simulink model "testing_control_with_feedback_estimate"  (Simulink 7.9)
settings: Solver=ode45  StartTime=0.0  StopTime=5  RelTol=1e-3
libraries: powerlib x6
settings Model: Creator=Dmitriy  LastModifiedBy=Dmitriy

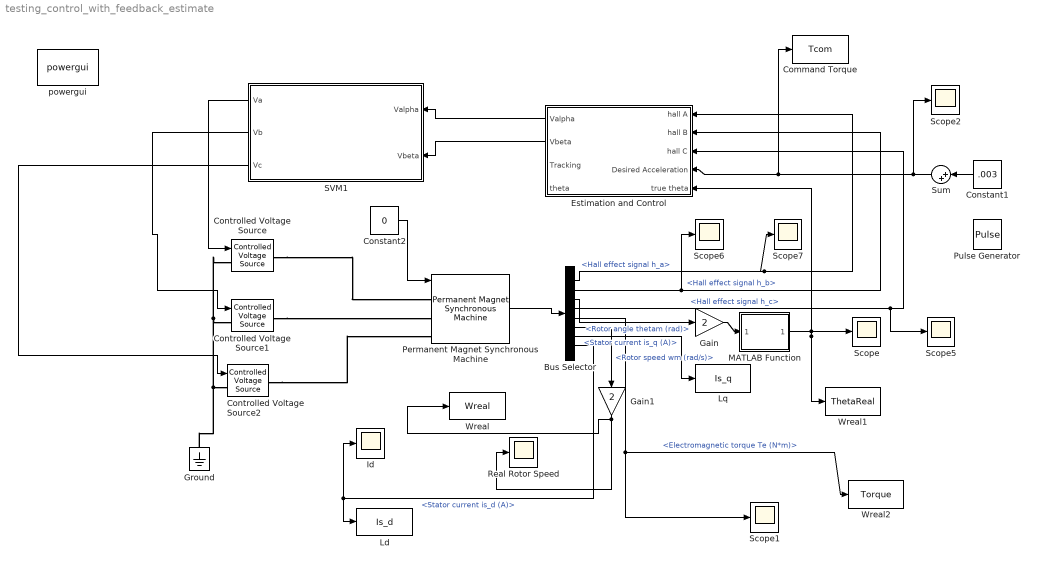
== system testing_control_with_feedback_estimate ==
  Bus Selector : BusSelector  OutputSignals=Hall effect signal h_a,Hall effect signal h_b,Hall effect signal h_c,Rotor angle thetam (rad),Electromagnetic torque Te (N*m),Rotor speed wm (rad/s),Stator current is_q (A),Stator current is_d (A)
  Command Torque : ToWorkspace  VariableName=Tcom  SampleTime=-1  SaveFormat=Timeseries
  Constant1 : Constant  Value=.003
  Constant2 : Constant  Value=0
  Controlled Voltage Source : powerlib/Electrical Sources/Controlled Voltage Source  Initialize=off  Source_Type=DC  Amplitude=0  Phase=0  Frequency=0  Measurements=None
  Controlled Voltage Source1 : powerlib/Electrical Sources/Controlled Voltage Source  Initialize=off  Source_Type=AC  Amplitude=0  Phase=0  Frequency=0  Measurements=None
  Controlled Voltage Source2 : powerlib/Electrical Sources/Controlled Voltage Source  Initialize=off  Source_Type=AC  Amplitude=0  Phase=0  Frequency=0  Measurements=None
  Estimation and Control : Subsystem  TreatAsAtomicUnit=on
  Gain : Gain  Gain=2
  Gain1 : Gain  Gain=2
  Ground : powerlib/Elements/Ground  LConnTagsString=a
  Id : Scope
      settings: YMin=-0.12  YMax=1.38778e-17  SaveName=ScopeData10
  Ld : ToWorkspace  VariableName=Is_d  SampleTime=-1  SaveFormat=Timeseries
  Lq : ToWorkspace  VariableName=Is_q  SampleTime=-1  SaveFormat=Timeseries
  MATLAB Function : MATLAB Function  TreatAsAtomicUnit=on
  Permanent Magnet Synchronous Machine : powerlib/Machines/Permanent Magnet Synchronous Machine  NbPhases=3  FluxDistribution=Sinusoidal  RotorType=Round  MechanicalLoad=Torque Tm  PresetModel=No  ShowDetailedParameters=on  Resistance=28.2  Inductance=8.5e-3  dqInductances=[0.006365 0.006365]  La=1940*10^-6  MachineConstant=Torque Constant (N.m / A_peak)  Flux=0.005225  VoltageCst=1.8954  TorqueCst=0.0181*sqrt(3)/2  Flat=120  Mechanical=[0.0001 1.35e-007 2 0]  PolePairs=2  InitialConditions=[2.5, 49.6, 0,0]  InitialConditions5ph=[0 0 0 0 0 0]  TsPowergui=0  TsBlock=-1  RefAngle=Aligned with phase A axis (original Park)
      link override From: GotoTag=tp895c948e_709d_4b9e_9e5d_f832b5ab97a5
  Pulse Generator : DiscretePulseGenerator  PulseType=Time based  Amplitude=-.006  Period=3  PulseWidth=50
  Real Rotor Speed : Scope
      settings: YMin=9.27  YMax=9.44  SaveName=ScopeData11
  SVM1 : Subsystem  TreatAsAtomicUnit=on  SystemSampleTime=.0001
  Scope{,1..2,5..7} (6 alike) : Scope
      Scope settings: YMin=0.03925  YMax=0.0396
      Scope1 settings: YMin=-1.1e+07  YMax=1.2e+07
      Scope2 settings: YMin=0.00317  YMax=0.00334  SaveName=ScopeData21
      Scope5 settings: SaveName=ScopeData5
      Scope6 settings: SaveName=ScopeData18
      Scope7 settings: SaveName=ScopeData20
  Sum : Sum  Inputs=|++
  Wreal : ToWorkspace  VariableName=Wreal  SampleTime=-1  SaveFormat=Timeseries
  Wreal1 : ToWorkspace  VariableName=ThetaReal  SampleTime=-1  SaveFormat=Timeseries
  Wreal2 : ToWorkspace  VariableName=Torque  SampleTime=-1  SaveFormat=Timeseries
  powergui : powerlib/powergui  Priority=1  SimulationMode=Continuous  SolverType=Tustin  SampleTime=50e-6  frequency=60  SPID=off  DisableSnubberDevices=off  DisableRonSwitches=off  DisableVfSwitches=off  SwTol=0  Interpol=off  DisplayEquations=off  FunctionMessages=off  frequencyindice=0  Pbase=100e6  ErrMax=1e-4  Iterations=50  UnitsV=kV  UnitsW=MW  echomessages=off  HookPort=off  EnableUseOfTLC=off  x0status=blocks  RestoreLinks=warning  ResistiveCurrentMeasurement=off  Ylog=off  Xlog=on  ShowGrid=off  save=off  variable=ZData  ZoomFFT=off  StartTime=0.0  cycles=1  DisplayStyle=1  FreqAxis=off  MaxFrequency=1000  frequencyindicesteady=1  display=off  methode=off
  wires:
  Permanent Magnet Synchronous Machine/1 -> Bus Selector/1
  Bus Selector/1 -> Estimation and Control/1(hall A), Scope7/1  "<Hall effect signal h_a>"
  Bus Selector/3 -> Estimation and Control/3(hall C), Scope5/1  "<Hall effect signal h_c>"
  Bus Selector/4 -> Gain/1  "<Rotor angle thetam (rad)>"
  Bus Selector/5 -> Wreal2/1, Scope1/1  "<Electromagnetic torque Te (N*m)>"
  Bus Selector/2 -> Estimation and Control/2(hall B), Scope6/1  "<Hall effect signal h_b>"
  Bus Selector/6 -> Gain1/1  "<Rotor speed wm (rad/s)>"
  MATLAB Function/1(lambda1) -> Wreal1/1, Scope/1, Estimation and Control/5(true theta)
  Gain/1 -> MATLAB Function/1(lambda)
  Constant2/1 -> Permanent Magnet Synchronous Machine/1
  Estimation and Control/1(Valpha) -> SVM1/1(Valpha)
  Estimation and Control/2(Vbeta) -> SVM1/2(Vbeta)
  Bus Selector/7 -> Lq/1  "<Stator current is_q (A)>"
  Bus Selector/8 -> Ld/1, Id/1  "<Stator current is_d (A)>"
  SVM1/1(Va) -> Controlled Voltage Source/1
  SVM1/2(Vb) -> Controlled Voltage Source1/1
  SVM1/3(Vc) -> Controlled Voltage Source2/1
  Constant1/1 -> Sum/1
  Sum/1 -> Scope2/1, Estimation and Control/4(Desired Acceleration), Command Torque/1
  Gain1/1 -> Real Rotor Speed/1, Wreal/1
  connections:
  Controlled Voltage Source2/LConn1 -- Controlled Voltage Source1/LConn1 -- Controlled Voltage Source/LConn1 -- Ground/LConn1
  Controlled Voltage Source/RConn1 -- Permanent Magnet Synchronous Machine/LConn1
  Controlled Voltage Source2/RConn1 -- Permanent Magnet Synchronous Machine/LConn3
  Controlled Voltage Source1/RConn1 -- Permanent Magnet Synchronous Machine/LConn2

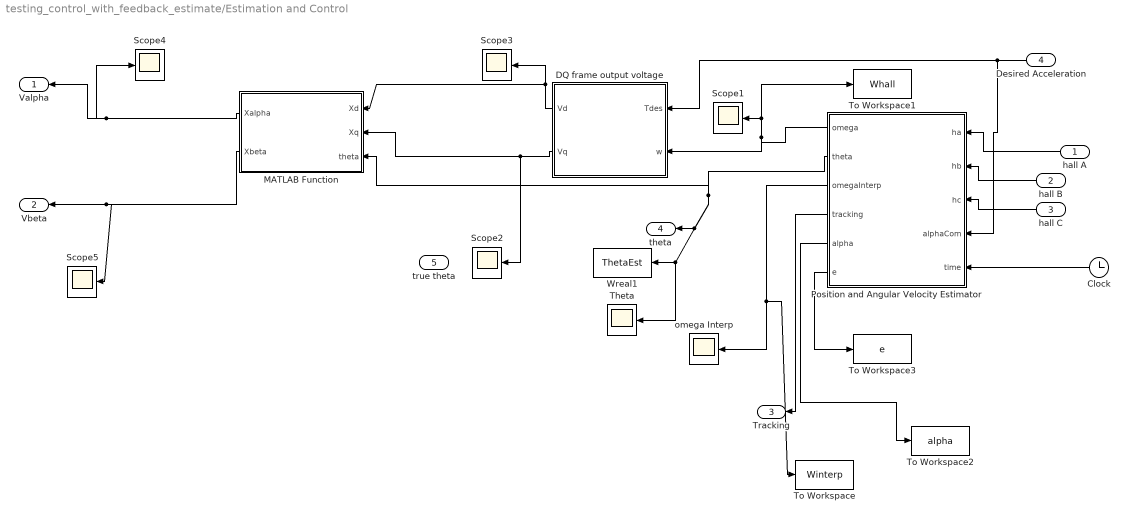
== system testing_control_with_feedback_estimate/Estimation and Control ==
  hall A : Inport
  hall B : Inport  Port=2
  hall C : Inport  Port=3
  Desired Acceleration : Inport  Port=4
  true theta : Inport  Port=5
  Clock : Clock
  DQ frame output voltage : MATLAB Function  TreatAsAtomicUnit=on
  MATLAB Function : MATLAB Function  TreatAsAtomicUnit=on
  Position and Angular Velocity Estimator : MATLAB Function  TreatAsAtomicUnit=on
  Scope{1..5} (5 alike) : Scope
      Scope1 settings: YMin=73.5  YMax=80  SaveName=ScopeData13
      Scope2 settings: YMin=4.44033  YMax=4.90773  SaveName=ScopeData14
      Scope3 settings: SaveName=ScopeData15
      Scope4 settings: SaveName=ScopeData16
      Scope5 settings: SaveName=ScopeData17
  Theta : Scope
      settings: YMin=0  YMax=6.5  SaveName=ScopeData12
  To Workspace : ToWorkspace  VariableName=Winterp  SampleTime=-1  SaveFormat=Timeseries
  To Workspace1 : ToWorkspace  VariableName=Whall  SampleTime=-1  SaveFormat=Timeseries
  To Workspace2 : ToWorkspace  VariableName=alpha  SampleTime=-1  SaveFormat=Timeseries
  To Workspace3 : ToWorkspace  VariableName=e  SampleTime=-1  SaveFormat=Timeseries
  Wreal1 : ToWorkspace  VariableName=ThetaEst  SampleTime=-1  SaveFormat=Timeseries
  omega Interp : Scope
      settings: YMin=0  YMax=3.25  SaveName=ScopeData19
  Valpha : Outport
  Vbeta : Outport  Port=2
  Tracking : Outport  Port=3
  theta : Outport  Port=4
  wires:
  Position and Angular Velocity Estimator/1(omega) -> Scope1/1, To Workspace1/1, DQ frame output voltage/2(w)
  Desired Acceleration/1 -> DQ frame output voltage/1(Tdes), Position and Angular Velocity Estimator/4(alphaCom)
  hall A/1 -> Position and Angular Velocity Estimator/1(ha)
  hall B/1 -> Position and Angular Velocity Estimator/2(hb)
  hall C/1 -> Position and Angular Velocity Estimator/3(hc)
  Position and Angular Velocity Estimator/2(theta) -> Theta/1, Wreal1/1, theta/1, MATLAB Function/3(theta)
  DQ frame output voltage/2(Vq) -> Scope2/1, MATLAB Function/2(Xq)
  DQ frame output voltage/1(Vd) -> Scope3/1, MATLAB Function/1(Xd)
  MATLAB Function/1(Xalpha) -> Valpha/1, Scope4/1
  MATLAB Function/2(Xbeta) -> Vbeta/1, Scope5/1
  Position and Angular Velocity Estimator/3(omegaInterp) -> omega Interp/1, To Workspace/1
  Clock/1 -> Position and Angular Velocity Estimator/5(time)
  Position and Angular Velocity Estimator/4(tracking) -> Tracking/1
  Position and Angular Velocity Estimator/5(alpha) -> To Workspace2/1
  Position and Angular Velocity Estimator/6(e) -> To Workspace3/1

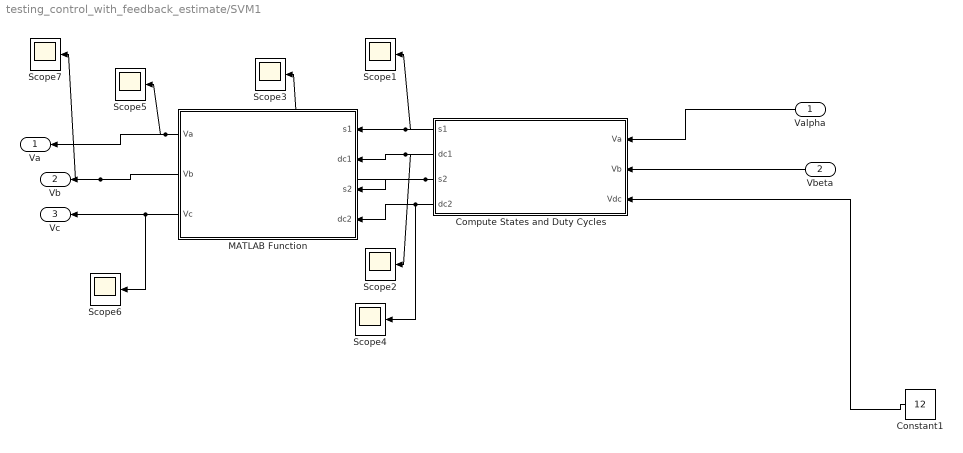
== system testing_control_with_feedback_estimate/SVM1 ==
  Valpha : Inport
  Vbeta : Inport  Port=2
  Compute States and Duty Cycles : MATLAB Function  TreatAsAtomicUnit=on
  Constant1 : Constant  Value=12
  MATLAB Function : MATLAB Function  TreatAsAtomicUnit=on
  Scope{1..7} (7 alike) : Scope
      Scope1 settings: SaveName=ScopeData6
      Scope2 settings: SaveName=ScopeData7
      Scope3 settings: SaveName=ScopeData8
      Scope4 settings: SaveName=ScopeData9
      Scope5 settings: SaveName=ScopeData2
      Scope6 settings: SaveName=ScopeData3
      Scope7 settings: SaveName=ScopeData4
  Va : Outport
  Vb : Outport  Port=2
  Vc : Outport  Port=3
  wires:
  Valpha/1 -> Compute States and Duty Cycles/1(Va)
  Vbeta/1 -> Compute States and Duty Cycles/2(Vb)
  Constant1/1 -> Compute States and Duty Cycles/3(Vdc)
  Compute States and Duty Cycles/1(s1) -> MATLAB Function/1(s1), Scope1/1
  Compute States and Duty Cycles/2(dc1) -> MATLAB Function/2(dc1), Scope2/1
  Compute States and Duty Cycles/3(s2) -> MATLAB Function/3(s2), Scope3/1
  Compute States and Duty Cycles/4(dc2) -> MATLAB Function/4(dc2), Scope4/1
  MATLAB Function/1(Va) -> Va/1, Scope5/1
  MATLAB Function/2(Vb) -> Vb/1, Scope7/1
  MATLAB Function/3(Vc) -> Vc/1, Scope6/1

== matlab function Estimation and Control/DQ frame output voltage ==
  data: Tdes input double; Vd output double; w input double; Vq output double
% function [Vd,Vq] = computeDQOutput(aDes,w, error)
% %#codegen
% %take the desired torque current 
% % speed and compute the output voltage vector in the DQ
% %frame. 
% Vd = 0;
% Vq = 0;
% coder.extrinsic('accelerationControl');
% 
% [Vd Vq] = accelerationControl(aDes,w,error);





function [Vd,Vq] = computeDQOutput(Tdes,w)
%#codegen
%take the desired torque current
% speed and compute the output voltage vector in the DQ
%frame.
w=w/2;
 L = 1940*10^-6; % with a factor of sqrt(3)/2 multiplying, Id rises with w
%also with no factor
%also divided by sqrt(3)
%also divided by 3
%also divided by 3*sqrt(3)

R = 28.2*sqrt(3)/2;
Kt = 18.1*10^-3*sqrt(3)/2; %Nm/Amp
Ke = Kt/sqrt(3);

%because I is assumed to be on Q axis, T = KtI
Ides = Tdes/Kt;

%bemf is on q axis
bemf = Ke*w;

%inductor impedance
ZL = L*w;

Vq = (bemf+Ides*R)*sqrt(3);
Vd = (-ZL*Ides)*sqrt(3);

== matlab function Estimation and Control/Position and Angular Velocity Estimator ==
  data: omega output double; ha input double; theta output double; hb input double; hc input double; alphaCom input double; omegaInterp output double; time input double; tracking output double; alpha output double; e output double
function [omega,theta, omegaInterp, tracking, alpha, e] = rotor_est(ha,hb,hc,alphaCom,time)
%#codegen

%estimate the position of the rotor in degrees electrical
%tracking is 0 or 1, 0 means the estimate is bad. Used for activating block
%commutation at initialization
omega=0;
theta=0;
omegaInterp = 0;
tracking = 0;
alpha = 0;
e =0;
coder.extrinsic('feedback_rotor_estimate');

[omega theta omegaInterp tracking alpha e] = feedback_rotor_estimate(ha,hb,hc,alphaCom,time);
end

== matlab function MATLAB Function ==
  data: lambda input double; lambda1 output double
function lambda1 = wrapTo2Pi(lambda)
%wrapTo2Pi Wrap angle in radians to [0 2*pi]
%
%   lambdaWrapped = wrapTo2Pi(LAMBDA) wraps angles in LAMBDA, in radians,
%   to the interval [0 2*pi] such that zero maps to zero and 2*pi maps
%   to 2*pi. (In general, positive multiples of 2*pi map to 2*pi and
%   negative multiples of 2*pi map to zero.)
%
%   See also wrapToPi, wrapTo180, wrapTo360.

% Copyright 2007-2008 The MathWorks, Inc.
% $Revision: 1.1.6.1 $  $Date: 2008/12/22 23:50:53 $


positiveInput = (lambda > 0);
lambda = mod(lambda, 2*pi);
lambda((lambda == 0) & positiveInput) = 2*pi;
lambda1=lambda;
end

== matlab function Estimation and Control/MATLAB Function ==
  data: Xd input double; Xalpha output double; Xq input double; theta input double; Xbeta output double
function [Xalpha,Xbeta] = inversePark(Xd,Xq,theta)
%#codegen
%implements inverse park as described in james mevey's thesis

c = cos(theta);
s = sin(theta);

ipm = [c -s; s c];

xab = ipm*[Xd Xq]';

Xalpha = xab(1);
Xbeta = xab(2);
end

== matlab function SVM1/Compute States and Duty Cycles ==
  data: Va input double; s1 output double; dc1 output double; Vb input double; s2 output double; Vdc input double; dc2 output double
function [s1,dc1, s2, dc2] = statesAndCycles(Va,Vb, Vdc)
%#codegen
    %Given desired Valpha and Vbeta, and the supply voltage, compute the inverter states to toggle
    %between and the duty cycle of each
    
    %right now we're saying that the length of each state vector is Vdc, which
    %is probably wrong
    
    ang = wrapTo2Pi(angle(Va+1i*Vb));
    
    sext = floor(ang/(pi/3));
    
    v1 = 1 +1i;
    v2 = 1 + 1i;
    
    %states as defined in james mevey's thesis
    %v1, v2 are complex values of the voltages
    switch sext
        case 0
            s1 = 1;
            v1 = Vdc;
            
            s2 = 2;
            [t1 t2] = pol2cart(pi/3,Vdc);
            v2 = t1+1i*t2;
            
        case 1
            s1 = 2;
            [t1 t2] = pol2cart(pi/3,Vdc);
            v1 = t1+1i*t2;
            
            s2 = 3;
            [t1 t2] = pol2cart(2*pi/3,Vdc);
            v2 = t1+1i*t2;
            
        case 2
            s1 = 3;
            [t1 t2] = pol2cart(2*pi/3,Vdc);
            v1 = t1+1i*t2;
            
            s2 = 4;
            [t1 t2] = pol2cart(pi,Vdc);
            v2 = t1+1i*t2;
        case 3
            s1 = 4;
            [t1 t2] = pol2cart(pi,Vdc);
            v1 = t1+1i*t2;
            
            s2 = 5;
            [t1 t2] = pol2cart(4*pi/3,Vdc);
            v2 = t1+1i*t2;
        case 4
            s1 = 5;
            [t1 t2] = pol2cart(4*pi/3,Vdc);
            v1 = t1+1i*t2;
            
            
            s2 = 6;
            [t1 t2] = pol2cart(5*pi/3,Vdc);
            v2 = t1+1i*t2;
        case 5
            s1 = 6;
            [t1 t2] = pol2cart(5*pi/3,Vdc);
            v1 = t1+1i*t2;
            
            s2 = 1;
            v2 = Vdc;
        otherwise
            s1 = 0;
            s2 = 0;
    end
    

num = Vb - imag(v1)*Va/real(v1);
den = imag(v2)-imag(v1)*real(v2)/real(v1);
dc2 = num/den;
dc1 = (Va - real(v2)*dc2)/real(v1);


    %solve for intersection of v1 line and v2 line translated to the desired
    %place
    
% 
%     num = Va-imag(v2)*Vb/real(v2)- imag(v1);
%     den = real(v1) - imag(v2)/real(v2);
%     
%     xint = num/den;
%     yint = (imag(v1)/real(v1))*xint;
%     
%     %duty cycle 1 equals length of sv1 divided by Vdc, which is nominal length
%     dc1 = sqrt(xint^2+yint^2)/Vdc;
%     
%     %duty cycle 2 is distance from the tip of sv1 to the desired point, divided
%     %by Vdc
%     
%     dc2 = sqrt((xint-Va)^2 +(yint - Vb)^2)/Vdc;

end

function lambda = wrapTo2Pi(lambda)
%wrapTo2Pi Wrap angle in radians to [0 2*pi]
%
%   lambdaWrapped = wrapTo2Pi(LAMBDA) wraps angles in LAMBDA, in radians,
%   to the interval [0 2*pi] such that zero maps to zero and 2*pi maps
%   to 2*pi. (In general, positive multiples of 2*pi map to 2*pi and
%   negative multiples of 2*pi map to zero.)
%
%   See also wrapToPi, wrapTo180, wrapTo360.

% Copyright 2007-2008 The MathWorks, Inc.
% $Revision: 1.1.6.1 $  $Date: 2008/12/22 23:50:53 $

positiveInput = (lambda > 0);
lambda = mod(lambda, 2*pi);
lambda((lambda == 0) & positiveInput) = 2*pi;
end

function p = angle(h)
%ANGLE  Phase angle.
%   ANGLE(H) returns the phase angles, in radians, of a matrix with
%   complex elements.
%
%   Class support for input X:
%      float: double, single
%
%   See also ABS, UNWRAP.

%   Copyright 1984-2010 The MathWorks, Inc.
%   $Revision: 5.7.4.2 $  $Date: 2010/04/21 21:31:19 $

p = atan2(imag(h), real(h));
end

== matlab function SVM1/MATLAB Function ==
  data: s1 input double; Va output double; dc1 input double; s2 input double; dc2 input double; Vb output double; Vc output double
function [Va,Vb,Vc] = PWM_module_inputs(s1,dc1,s2,dc2)
%#codegen
%given the two states to switch between and the duty cycle of each, compute
%the proper duty cycles and phases for each leg of the half bridge. Duty
%cycles should be between 1 and 1000, as should phases. If duty cycle is
%1000, and phase is 400, then the duty cycle really only ends up being 400,
%get it? If not, look at the pwm block.

%pattern is: all low, then s1, then s2
dc=[0 0 0];

switch(s1)
    
    case 1
        if(s2==2)
            dc=[dc1+dc2 dc2 0];
        else
            dc = [dc1+dc2 0 dc2];
        end
    case 2
        if(s2==3)
            dc = [dc1 dc1+dc2 0];
        else
            dc = [dc1+dc2 dc1 0];
        end
    case 3
        if(s2==4)
            dc = [0 dc1+dc2 dc2];
        else
            dc = [dc2 dc1+dc2 0];
        end
    case 4
        if(s2 == 5)
            dc = [0 dc1 dc1+dc2];
        else
            dc = [0 dc1+dc2 dc1]
        end
    case 5
        if(s2==6)
            dc = [dc2 0 dc1+dc2];
        else
            dc= [0 dc2 dc1+dc2];
        end
    case 6
        
        if(s2==1)
            dc = [dc1+dc2 0 dc1];
        else
            dc = [dc1 0 dc1+dc2]
        end
    otherwise
        
end
Va = dc(1)*12;
Vb = dc(2)*12;
Vc = dc(3)*12;

end
